simulink model "thermostat_task"  (Simulink 3.00)
libraries: mathlib x2, arclib x2, analoglib x1

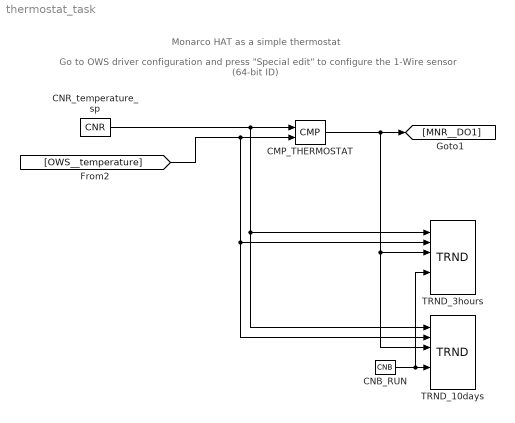
== system thermostat_task ==
  note: Go to OWS driver configuration and press "Special edit" to configure the 1-Wire sensor (64-bit ID)
  note: Monarco HAT as a simple thermostat
  CMP_THERMOSTAT : analoglib/CMP  hys=0.5
  CNB_RUN : mathlib/CNB  YCN=on
  CNR_temperature_sp : mathlib/CNR  ycn=21.8
  TRND_10days : arclib/TRND  n=4  l=86400  btype=8: Double  ptype1=1: Store  ptype2=1: Store  ptype3=1: Store  ptype4=1: Store  pfac=20  afac=0  arc=0  id=1  Title=Thermostat actions (10 days)  timesrc=1
  TRND_3hours : arclib/TRND  n=4  l=10800  btype=8: Double  ptype1=1: Store  ptype2=1: Store  ptype3=1: Store  ptype4=1: Store  pfac=2  afac=0  arc=0  id=1  Title=Thermostat actions (3 hours)  timesrc=1
  wires:
  CMP_THERMOSTAT/1 -> [MNR__DO1], TRND_10days/3, TRND_3hours/3
  CNB_RUN/1 -> TRND_10days/5, TRND_3hours/5
  CNR_temperature_sp/1 -> CMP_THERMOSTAT/1, TRND_10days/1, TRND_3hours/1
  [OWS__temperature] -> CMP_THERMOSTAT/2, TRND_10days/2, TRND_3hours/2
